simulink model "Feeder_IREQ_2012"  (Simulink 8.3)
settings: Solver=FixedStepDiscrete  StartTime=0.0  StopTime=100  FixedStep=50e-6  RelTol=1e-3
InitFcn:
  | Ts= 50e-6;
undefined symbols (not defined in the file): D11, Delta, DiscIntNeverNeededParam, Ion, kaimal_num, Lithium, u0
libraries: powerlib x62, powerlib_extras x49, simulink x14, simulink_extras x12, sps_avr x2, electricdrivelib x1
(part 3 of 5)

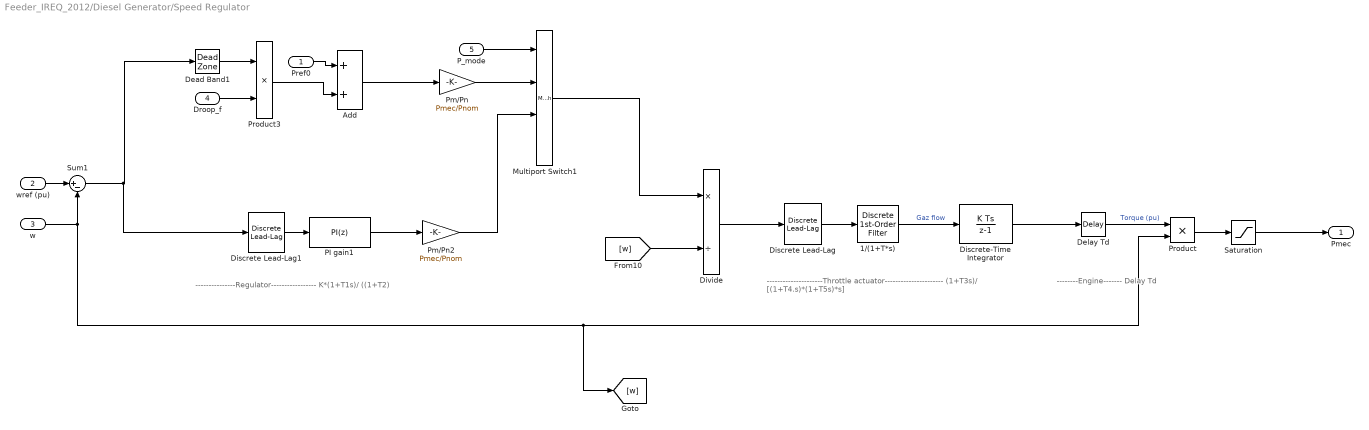
== system Feeder_IREQ_2012/Diesel Generator/Speed Regulator ==
  note: ---------------------Throttle actuator----------------------
      | (1+T3s)/ [(1+T4.s)*(1+T5s)*s]
  note: ---------------Regulator-----------------
      | K*(1+T1s)/ ((1+T2)
  note: --------Engine-------
      | Delay Td
  Pref0 : Inport
  wref (pu) : Inport  Port=2
  w : Inport  Port=3
  Droop_f : Inport  Port=4
  P_mode : Inport  Port=5
  1/(1+T*s) : powerlib_extras/Discrete  Control Blocks/Discrete 1st-Order Filter  FilterType=Lowpass  Tc=Ta(3)  Ts=Ts  Initialize=off  Vac_Init=[0.8 -25 60]  Vdc_Init=-0.4  PlotResponse=off  param1=[1 500 0.1]
  Add : Sum
  Dead Band1 : DeadZone  LowerValue=-0.001  UpperValue=0.001  SaturateOnIntegerOverflow=on
  Delay Td : TransportDelay  DelayTime=Td  InitialOutput=Pm0
  Discrete Lead-Lag : powerlib_extras/Discrete  Control Blocks/Discrete Lead-Lag  T1=Ta(1)  T2=Ta(2)  V_Init=0  Ts=Ts
  Discrete Lead-Lag1 : powerlib_extras/Discrete  Control Blocks/Discrete Lead-Lag  T1=Tr(1)  T2=Tr(2)  V_Init=0  Ts=Ts
  Discrete-Time Integrator : DiscreteIntegrator  InitialCondition=Pm0  SampleTime=Ts  LimitOutput=on  UpperSaturationLimit=Tlim(2)  LowerSaturationLimit=Tlim(1)  ICPrevOutput=DiscIntNeverNeededParam  ICPrevScaledInput=DiscIntNeverNeededParam
  Divide : Product  Inputs=*/
  Multiport Switch1 : MultiPortSwitch  SaturateOnIntegerOverflow=on  InputSameDT=on
  PI gain1 : simulink/Continuous/PID Controller  Controller=PI  TimeDomain=Discrete-time  SampleTime=-1  IntegratorMethod=Forward Euler  FilterMethod=Forward Euler  Form=Parallel  P=100  I=100  D=-14.7932376623781  N=587.187356380874  InitialConditionSource=internal  InitialConditionForIntegrator=0  InitialConditionForFilter=0  ExternalReset=none  LimitOutput=off  UpperSaturationLimit=1.05  LowerSaturationLimit=.95  LinearizeAsGain=off  AntiWindupMode=back-calculation  Kb=1  TrackingMode=off  Kt=1  PParamMin=[]  PParamMax=[]  IParamMin=[]  IParamMax=[]  DParamMin=[]  DParamMax=[]  NParamMin=[]  NParamMax=[]  KbParamMin=[]  KbParamMax=[]  KtParamMin=[]  KtParamMax=[]  POutMin=[]  POutMax=[]  IOutMin=[]  IOutMax=[]  DOutMin=[]  DOutMax=[]  NOutMin=[]  NOutMax=[]  KbOutMin=[]  KbOutMax=[]  KtOutMin=[]  KtOutMax=[]  IntegratorOutMin=[]  IntegratorOutMax=[]  FilterOutMin=[]  FilterOutMax=[]  SumOutMin=[]  SumOutMax=[]  SumI1OutMin=[]  SumI1OutMax=[]  SumI2OutMin=[]  SumI2OutMax=[]  SumI3OutMin=[]  SumI3OutMax=[]  SumDOutMin=[]  SumDOutMax=[]  SaturationOutMin=[]  SaturationOutMax=[]  IntegratorContinuousStateAttributes=''  IntegratorStateMustResolveToSignalObject=off  IntegratorRTWStateStorageClass=Auto  FilterContinuousStateAttributes=''  FilterStateMustResolveToSignalObject=off  FilterRTWStateStorageClass=Auto
  Pm/Pn : Gain  Gain=Pmec/Pnom
  Pm/Pn2 : Gain  Gain=Pmec/Pnom
  Product : Product  SaturateOnIntegerOverflow=on  InputSameDT=on  OutDataTypeStr=Inherit: Same as first input
  Product3 : Product  RndMeth=Zero
  Saturation : Saturate  UpperLimit=Pmec/Pnom  LowerLimit=0
  Sum1 : Sum  Inputs=|+-  SaturateOnIntegerOverflow=on
  Pmec : Outport  InitialOutput=0
  wires:
  wref (pu)/1 -> Sum1/1
  Dead Band1/1 -> Product3/1
  Droop_f/1 -> Product3/2
  Pref0/1 -> Add/1
  Product3/1 -> Add/2
  P_mode/1 -> Multiport Switch1/1
  Add/1 -> Pm/Pn/1
  Pm/Pn/1 -> Multiport Switch1/2
  w/1 -> [w], Product/2, Sum1/2
  Sum1/1 -> Discrete Lead-Lag1/1, Dead Band1/1
  Delay Td/1 -> Product/1  "Torque (pu)"
  Discrete Lead-Lag/1 -> 1/(1+T*s)/1
  1/(1+T*s)/1 -> Discrete-Time Integrator/1  "Gaz flow"
  Discrete Lead-Lag1/1 -> PI gain1/1
  Discrete-Time Integrator/1 -> Delay Td/1
  PI gain1/1 -> Pm/Pn2/1
  [w] -> Divide/2
  Divide/1 -> Discrete Lead-Lag/1
  Saturation/1 -> Pmec/1
  Product/1 -> Saturation/1
  Multiport Switch1/1 -> Divide/1
  Pm/Pn2/1 -> Multiport Switch1/3

== system Feeder_IREQ_2012/Diesel Generator/Voltage Droop with Q ==
  Vref : Inport
  Droop_v : Inport  Port=2
  fixed_Q : Inport  Port=3
  Qpcc : Inport  Port=4
  VPCC : Inport  Port=5
  Dead Band1 : DeadZone  LowerValue=-0.01  UpperValue=0.01  SaturateOnIntegerOverflow=on
  PI1 : simulink/Continuous/PID Controller  Controller=PI  TimeDomain=Discrete-time  SampleTime=-1  IntegratorMethod=Forward Euler  FilterMethod=Forward Euler  Form=Parallel  P=.5  I=5  D=-14.7932376623781  N=587.187356380874  InitialConditionSource=internal  InitialConditionForIntegrator=0  InitialConditionForFilter=0  ExternalReset=none  LimitOutput=on  UpperSaturationLimit=1.05  LowerSaturationLimit=.94  LinearizeAsGain=off  AntiWindupMode=none  Kb=1  TrackingMode=off  Kt=1  PParamMin=[]  PParamMax=[]  IParamMin=[]  IParamMax=[]  DParamMin=[]  DParamMax=[]  NParamMin=[]  NParamMax=[]  KbParamMin=[]  KbParamMax=[]  KtParamMin=[]  KtParamMax=[]  POutMin=[]  POutMax=[]  IOutMin=[]  IOutMax=[]  DOutMin=[]  DOutMax=[]  NOutMin=[]  NOutMax=[]  KbOutMin=[]  KbOutMax=[]  KtOutMin=[]  KtOutMax=[]  IntegratorOutMin=[]  IntegratorOutMax=[]  FilterOutMin=[]  FilterOutMax=[]  SumOutMin=[]  SumOutMax=[]  SumI1OutMin=[]  SumI1OutMax=[]  SumI2OutMin=[]  SumI2OutMax=[]  SumI3OutMin=[]  SumI3OutMax=[]  SumDOutMin=[]  SumDOutMax=[]  SaturationOutMin=[]  SaturationOutMax=[]  IntegratorContinuousStateAttributes=''  IntegratorStateMustResolveToSignalObject=off  IntegratorRTWStateStorageClass=Auto  FilterContinuousStateAttributes=''  FilterStateMustResolveToSignalObject=off  FilterRTWStateStorageClass=Auto
  Product3 : Product  RndMeth=Zero
  Sum1 : Sum  Inputs=+-  SaturateOnIntegerOverflow=on  InputSameDT=on  OutDataTypeStr=Inherit: Same as first input
  Sum2 : Sum  Inputs=+-  SaturateOnIntegerOverflow=on  InputSameDT=on  OutDataTypeStr=Inherit: Same as first input
  Sum4 : Sum  SaturateOnIntegerOverflow=on  InputSameDT=on  OutDataTypeStr=Inherit: Same as first input
  Vf : Outport
  wires:
  Sum2/1 -> Dead Band1/1
  Dead Band1/1 -> Product3/1
  Droop_v/1 -> Product3/2
  Product3/1 -> Sum4/1
  Vref/1 -> Sum2/1
  Qpcc/1 -> Sum1/2
  Sum1/1 -> PI1/1
  PI1/1 -> Vf/1
  fixed_Q/1 -> Sum4/2
  Sum4/1 -> Sum1/1
  VPCC/1 -> Sum2/2

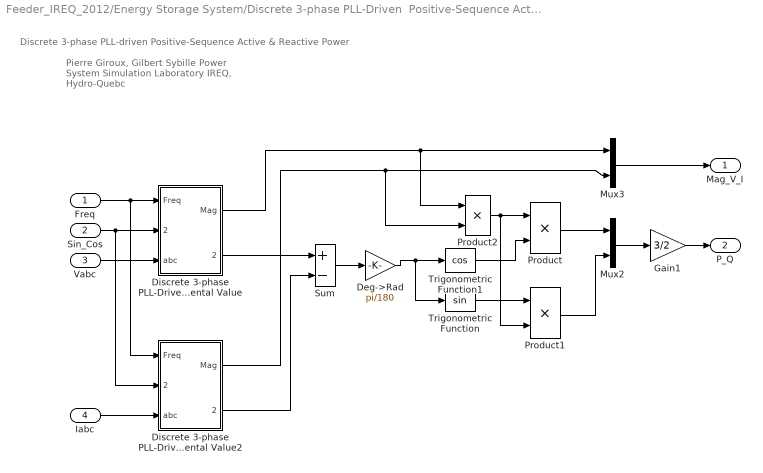
== system Feeder_IREQ_2012/Energy Storage System/Discrete 3-phase PLL-Driven  Positive-Sequence Active & Reactive Power ==
  note: Pierre Giroux, Gilbert Sybille
      | Power System Simulation Laboratory
      | IREQ, Hydro-Quebc
  note: Discrete 3-phase PLL-driven Positive-Sequence Active & Reactive Power
  Freq : Inport  PortDimensions=1
  Sin_Cos : Inport  Port=2  PortDimensions=2
  Vabc : Inport  Port=3  PortDimensions=3
  Iabc : Inport  Port=4  PortDimensions=3
  Deg->Rad : Gain  Gain=pi/180  SaturateOnIntegerOverflow=on  OutDataTypeStr=Inherit: Same as input  ParamDataTypeStr=Inherit: Same as input
  Discrete 3-phase PLL-Driven Positive-Sequence Fundamental Value : Subsystem  mask(Discrete 3-phase PLL-Driven Positive-Sequence Fundamental Value){Finit=Finit, Fmin=Fmin, Par_Init=Par_Vinit, Ts=Ts}
      mask prompts: Finit "Initial frequency (Hz):"; Fmin "Minimum frequency (Hz):"; Par_Init "Initial input (positive component): [ Mag  Phase-relative-to-PLL(degrees) ]"; Ts "Sample time:"
      mask help:
      | For a supplied fundamental frequency (port Freq), this discrete block computes  the positive-sequence component (Magnitude and Phase)  of a set of three balanced or unbalanced signals (port abc) which may contain harmonics.
      |  Input port "Sin_Cos" (a two-dimension signal) provides the reference frame required for the computation..
      |  First and second outputs return respectively the magnitude and phase (in degrees relative to the PLL phase)) of the fundamental.
      | For the first cycle of simulation, the outputs are held constant to the values specified by the parameter "Initial input".
      | constant to the values specified by the parameter "Initial input". The value of the parameter "Minimum frequency" is used to determine the buffer size of the "Variable Transport Delay" block found inside this subsystem.
      mask init:
      | Real_Init=Par_Init(1)*cos(pi/180*Par_Init(2));
      | Imag_Init=Par_Init(1)*sin(pi/180*Par_Init(2));
      | power_initmask();
      settings: OpenFcn=power_openblockproxy();
  Discrete 3-phase PLL-Driven Positive-Sequence Fundamental Value2 : Subsystem  mask(Discrete 3-phase PLL-Driven Positive-Sequence Fundamental Value){Finit=Finit, Fmin=Fmin, Par_Init=Par_Iinit, Ts=Ts}
      mask prompts: Finit "Initial frequency (Hz):"; Fmin "Minimum frequency (Hz):"; Par_Init "Initial input (positive component): [ Mag  Phase-relative-to-PLL(degrees) ]"; Ts "Sample time:"
      mask help:
      | For a supplied fundamental frequency (port Freq), this discrete block computes  the positive-sequence component (Magnitude and Phase)  of a set of three balanced or unbalanced signals (port abc) which may contain harmonics.
      |  Input port "Sin_Cos" (a two-dimension signal) provides the reference frame required for the computation..
      |  First and second outputs return respectively the magnitude and phase (in degrees relative to the PLL phase)) of the fundamental.
      | For the first cycle of simulation, the outputs are held constant to the values specified by the parameter "Initial input".
      | constant to the values specified by the parameter "Initial input". The value of the parameter "Minimum frequency" is used to determine the buffer size of the "Variable Transport Delay" block found inside this subsystem.
      mask init:
      | Real_Init=Par_Init(1)*cos(pi/180*Par_Init(2));
      | Imag_Init=Par_Init(1)*sin(pi/180*Par_Init(2));
      | power_initmask();
      settings: OpenFcn=power_openblockproxy();
  Gain1 : Gain  Gain=3/2  SaturateOnIntegerOverflow=on  OutDataTypeStr=Inherit: Same as input  ParamDataTypeStr=Inherit: Same as input
  Mux2 : Mux  Inputs=2
  Mux3 : Mux  Inputs=2
  Product : Product  SaturateOnIntegerOverflow=on  InputSameDT=on  OutDataTypeStr=Inherit: Same as first input
  Product1 : Product  SaturateOnIntegerOverflow=on  InputSameDT=on  OutDataTypeStr=Inherit: Same as first input
  Product2 : Product  SaturateOnIntegerOverflow=on  InputSameDT=on  OutDataTypeStr=Inherit: Same as first input
  Sum : Sum  Inputs=+-  SaturateOnIntegerOverflow=on  InputSameDT=on  OutDataTypeStr=Inherit: Same as first input
  Trigonometric Function : Trigonometry
  Trigonometric Function1 : Trigonometry  Operator=cos
  Mag_V_I : Outport
  P_Q : Outport  Port=2
  wires:
  Iabc/1 -> Discrete 3-phase PLL-Driven Positive-Sequence Fundamental Value2/3(abc)
  Discrete 3-phase PLL-Driven Positive-Sequence Fundamental Value2/1(Mag) -> Product2/2, Mux3/2
  Product2/1 -> Product1/2, Product/1
  Gain1/1 -> P_Q/1
  Mux3/1 -> Mag_V_I/1
  Product1/1 -> Mux2/2
  Product/1 -> Mux2/1
  Mux2/1 -> Gain1/1
  Trigonometric Function/1 -> Product1/1
  Trigonometric Function1/1 -> Product/2
  Deg->Rad/1 -> Trigonometric Function/1, Trigonometric Function1/1
  Sum/1 -> Deg->Rad/1
  Discrete 3-phase PLL-Driven Positive-Sequence Fundamental Value2/2(Phase) -> Sum/2
  Discrete 3-phase PLL-Driven Positive-Sequence Fundamental Value/1(Mag) -> Product2/1, Mux3/1
  Discrete 3-phase PLL-Driven Positive-Sequence Fundamental Value/2(Phase) -> Sum/1
  Sin_Cos/1 -> Discrete 3-phase PLL-Driven Positive-Sequence Fundamental Value2/2(Sin_Cos), Discrete 3-phase PLL-Driven Positive-Sequence Fundamental Value/2(Sin_Cos)
  Freq/1 -> Discrete 3-phase PLL-Driven Positive-Sequence Fundamental Value2/1(Freq), Discrete 3-phase PLL-Driven Positive-Sequence Fundamental Value/1(Freq)
  Vabc/1 -> Discrete 3-phase PLL-Driven Positive-Sequence Fundamental Value/3(abc)

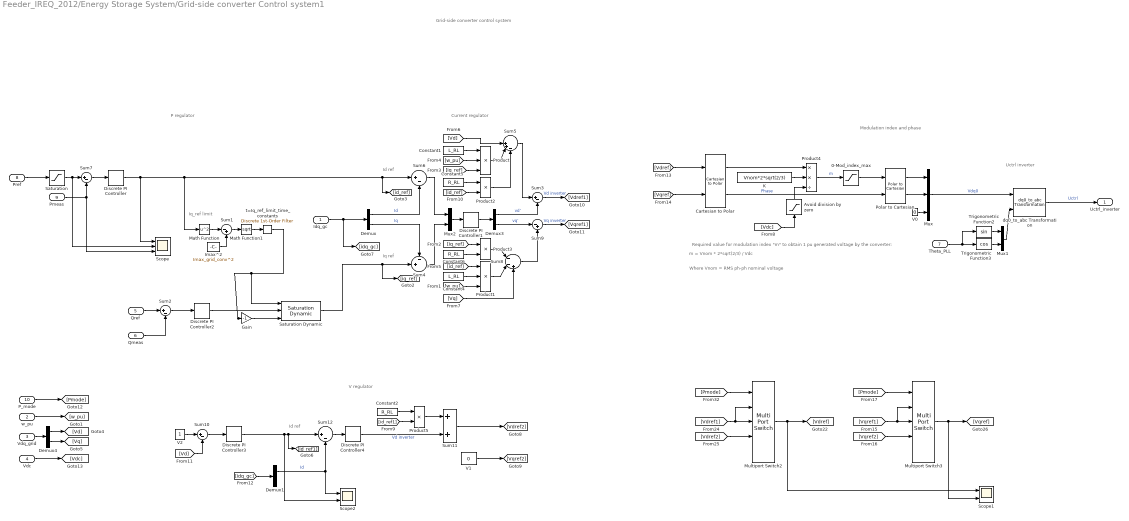
== system Feeder_IREQ_2012/Energy Storage System/Grid-side converter Control system1 ==
  note: Grid-side converter control system
  note: P regulator
  note: Iq_ref limit
  note: Current regulator
  note: Id ref
  note: Iq ref
  note: Required value for modulation index "m" to obtain 1 pu generated voltage by the converter:
  note: m = Vnom * 2*sqrt(2/3) / Vdc
  note: Where Vnom = RMS ph-ph nominal voltage
  note: Modulation index and phase
  note: Uctrl inverter
  note: V regulator
  note: Id ref
  Idq_gc : Inport
  w_pu : Inport  Port=2
  Vdq_grid : Inport  Port=3
  Vdc : Inport  Port=4
  Qref : Inport  Port=5
  Qmeas : Inport  Port=6
  Theta_PLL : Inport  Port=7
  Pref : Inport  Port=8
  Pmeas : Inport  Port=9
  P_mode : Inport  Port=10
  0-Mod_index_max : Saturate  UpperLimit=Mod_index_max  LowerLimit=0
  Avoid division by zero : Saturate  UpperLimit=1e6  LowerLimit=1e-6
  Cartesian to Polar : simulink_extras/Transformations/Cartesian to Polar
  Constant1 : Constant  Value=L_RL
  Constant2 : Constant  Value=R_RL
  Constant4 : Constant  Value=L_RL
  Constant5 : Constant  Value=R_RL
  Constant6 : Constant  Value=R_RL
  Demux{,1,3..4} (4 alike) : Demux  Outputs=2
  Discrete PI Controller : powerlib_extras/Discrete  Control Blocks/Discrete PI Controller  Kp=1  Ki=50  Par_Limits=[1 -1]*Imax_grid_conv  Init=0  Ts=Ts
  Discrete PI Controller1 : powerlib_extras/Discrete  Control Blocks/Discrete PI Controller  Kp=1  Ki=50  Par_Limits=[1 -1]*Current_reg_output_limit  Init=0  Ts=Ts
  Discrete PI Controller2 : powerlib_extras/Discrete  Control Blocks/Discrete PI Controller  Kp=1  Ki=50  Par_Limits=[1 -1]*Imax_grid_conv  Init=0  Ts=Ts
  Discrete PI Controller3 : powerlib_extras/Discrete  Control Blocks/Discrete PI Controller  Kp=1  Ki=10  Par_Limits=[1 -1]*Imax_grid_conv  Init=0  Ts=Ts
  Discrete PI Controller4 : powerlib_extras/Discrete  Control Blocks/Discrete PI Controller  Kp=1  Ki=50  Par_Limits=[1 -1]*Current_reg_output_limit  Init=0  Ts=Ts
  Gain : Gain  Gain=-1  SaturateOnIntegerOverflow=on  OutDataTypeStr=Inherit: Same as input  ParamDataTypeStr=Inherit: Same as input
  Imax^2 : Constant  Value=Imax_grid_conv^2
  K : Constant  Value=Vnom*2*sqrt(2/3)
  Math Function : Math  Operator=square  SaturateOnIntegerOverflow=on
  Math Function1 : Math  Operator=sqrt  SaturateOnIntegerOverflow=on
  Multiport Switch2 : MultiPortSwitch  Inputs=4  SaturateOnIntegerOverflow=on  InputSameDT=on
  Multiport Switch3 : MultiPortSwitch  Inputs=4  SaturateOnIntegerOverflow=on  InputSameDT=on
  Mux : Mux  Inputs=3
  Mux1 : Mux  Inputs=2
  Mux2 : Mux  Inputs=2
  Polar to Cartesian : simulink_extras/Transformations/Polar to Cartesian
  Product : Product  Inputs=3  SaturateOnIntegerOverflow=on  InputSameDT=on  OutDataTypeStr=Inherit: Same as first input
  Product1 : Product  Inputs=3  SaturateOnIntegerOverflow=on  InputSameDT=on  OutDataTypeStr=Inherit: Same as first input
  Product2 : Product  SaturateOnIntegerOverflow=on  InputSameDT=on  OutDataTypeStr=Inherit: Same as first input
  Product3 : Product  SaturateOnIntegerOverflow=on  InputSameDT=on  OutDataTypeStr=Inherit: Same as first input
  Product4 : Product  Inputs=**/  SaturateOnIntegerOverflow=on  InputSameDT=on  OutDataTypeStr=Inherit: Same as first input
  Product5 : Product  SaturateOnIntegerOverflow=on  InputSameDT=on  OutDataTypeStr=Inherit: Same as first input
  Saturation : Saturate  UpperLimit=Pbat/Pnom  LowerLimit=-Pbat/Pnom
  Saturation Dynamic : simulink/Discontinuities/Saturation Dynamic  OutMin=[]  OutMax=[]  OutDataTypeStr=Inherit: Same as second input  OutDataType=fixdt(1, 16)  OutScaling=2^-10  DoSatur=off
  Scope : Scope  NumInputPorts=3
  Scope1 : Scope  NumInputPorts=2
  Scope2 : Scope  NumInputPorts=2
  Sum1 : Sum  Inputs=|-+  SaturateOnIntegerOverflow=on  InputSameDT=on  OutDataTypeStr=Inherit: Same as first input
  Sum{2..3,6..7,10,12} (6 alike) : Sum  Inputs=|+-  SaturateOnIntegerOverflow=on  InputSameDT=on  OutDataTypeStr=Inherit: Same as first input
  Sum11 : Sum  SaturateOnIntegerOverflow=on  InputSameDT=on  OutDataTypeStr=Inherit: Same as first input
  Sum4 : Sum  Inputs=-+|  SaturateOnIntegerOverflow=on  InputSameDT=on  OutDataTypeStr=Inherit: Same as first input
  Sum5 : Sum  Inputs=||++-  SaturateOnIntegerOverflow=on  InputSameDT=on  OutDataTypeStr=Inherit: Same as first input
  Sum8 : Sum  Inputs=|--+  SaturateOnIntegerOverflow=on  InputSameDT=on  OutDataTypeStr=Inherit: Same as first input
  Sum9 : Sum  Inputs=|-+  SaturateOnIntegerOverflow=on  InputSameDT=on  OutDataTypeStr=Inherit: Same as first input
  Trigonometric Function2 : Trigonometry
  Trigonometric Function3 : Trigonometry  Operator=cos
  V0 : Constant  Value=0
  V1 : Constant  Value=0
  V2 : Constant
  dq0_to_abc Transformation : powerlib_extras/Measurements/dq0_to_abc Transformation
  t=Iq_ref_limit_time_constants : powerlib_extras/Discrete  Control Blocks/Discrete 1st-Order Filter  FilterType=Lowpass  Tc=Iq_ref_limit_time_constant  Ts=Ts  Initialize=on  Vac_Init=[0 0 0]  Vdc_Init=Imax_grid_conv  PlotResponse=off  param1=[1 500 0.1]
  Uctrl_inverter : Outport
  wires:
  Vdc/1 -> [Vdc]
  Vdq_grid/1 -> Demux4/1
  Discrete PI Controller/1 -> Math Function/1, Sum6/1, [id_ref], Scope/1
  Qmeas/1 -> Sum2/2
  Sum2/1 -> Discrete PI Controller2/1
  Math Function1/1 -> t=Iq_ref_limit_time_constants/1
  Sum1/1 -> Math Function1/1
  Imax^2/1 -> Sum1/2
  Math Function/1 -> Sum1/1
  t=Iq_ref_limit_time_constants/1 -> Gain/1, Saturation Dynamic/1
  Constant4/1 -> Product1/2
  Discrete PI Controller1/1 -> Demux3/1
  Mux2/1 -> Discrete PI Controller1/1
  Constant1/1 -> Product/1
  Demux/2 -> Sum4/1  "Iq"
  Demux/1 -> Sum6/2  "Id"
  Product/1 -> Sum5/2
  Constant5/1 -> Product2/1
  Constant6/1 -> Product3/2
  Product1/1 -> Sum8/2
  Product2/1 -> Sum5/3
  Product3/1 -> Sum8/1
  Sum6/1 -> Mux2/1
  Sum4/1 -> Mux2/2
  [w_pu] -> Product1/3
  [w_pu] -> Product/2
  [iq_ref] -> Product/3
  [id_ref] -> Product2/2
  [iq_ref] -> Product3/1
  [id_ref] -> Product1/1
  Demux3/1 -> Sum3/2  "vd'"
  Demux3/2 -> Sum9/1  "vq'"
  w_pu/1 -> [w_pu]
  Demux4/1 -> [Vd]
  Demux4/2 -> [Vq]
  [Vq] -> Sum8/3
  [Vd] -> Sum5/1
  Product4/1 -> 0-Mod_index_max/1  "m"
  K/1 -> Product4/2
  Avoid division by zero/1 -> Product4/3
  Cartesian to Polar/1 -> Product4/1
  [Vdc] -> Avoid division by zero/1
  Polar to Cartesian/2 -> Mux/2
  Polar to Cartesian/1 -> Mux/1
  V0/1 -> Mux/3
  Trigonometric Function3/1 -> Mux1/2
  Trigonometric Function2/1 -> Mux1/1
  Mux1/1 -> dq0_to_abc Transformation/2
  Cartesian to Polar/2 -> Polar to Cartesian/2  "Phase"
  Mux/1 -> dq0_to_abc Transformation/1  "Vdq0"
  dq0_to_abc Transformation/1 -> Uctrl_inverter/1  "Uctrl"
  Idq_gc/1 -> [idq_gc], Demux/1
  0-Mod_index_max/1 -> Polar to Cartesian/1
  Sum5/1 -> Sum3/1
  Sum8/1 -> Sum9/2
  Pref/1 -> Saturation/1
  Qref/1 -> Sum2/1
  Gain/1 -> Saturation Dynamic/3
  Discrete PI Controller2/1 -> Saturation Dynamic/2
  Pmeas/1 -> Scope/3, Sum7/2
  Saturation Dynamic/1 -> Sum4/2, [iq_ref]
  Saturation/1 -> Scope/2, Sum7/1
  Sum7/1 -> Discrete PI Controller/1
  Theta_PLL/1 -> Trigonometric Function2/1, Trigonometric Function3/1
  Discrete PI Controller3/1 -> Scope2/2, Sum12/1, [id_ref1]
  Demux1/1 -> Scope2/1, Sum12/2  "Id"
  Constant2/1 -> Product5/1
  Sum12/1 -> Discrete PI Controller4/1
  [id_ref1] -> Product5/2
  Discrete PI Controller4/1 -> Sum11/2  "Vd inverter"
  V2/1 -> Sum10/1
  Sum10/1 -> Discrete PI Controller3/1
  [Vd] -> Sum10/2
  Sum11/1 -> [Vdref2]
  Product5/1 -> Sum11/1
  [idq_gc] -> Demux1/1
  [Pmode] -> Multiport Switch2/1
  [Pmode] -> Multiport Switch3/1
  Multiport Switch2/1 -> Scope1/1, [Vdref]
  Multiport Switch3/1 -> Scope1/2, [Vqref]
  V1/1 -> [Vqref2]
  Sum3/1 -> [Vdref1]  "Vd inverter"
  Sum9/1 -> [Vqref1]  "Vq inverter"
  P_mode/1 -> [Pmode]
  [Vqref2] -> Multiport Switch3/4
  [Vdref1] -> Multiport Switch2/2, Multiport Switch2/3
  [Vdref2] -> Multiport Switch2/4
  [Vqref1] -> Multiport Switch3/2, Multiport Switch3/3
  [Vdref] -> Cartesian to Polar/1
  [Vqref] -> Cartesian to Polar/2

== system Feeder_IREQ_2012/Energy Storage System/Reactive power gain1 ==
  In1 : Inport
  Product : Product  RndMeth=Zero
  Product1 : Product  RndMeth=Zero
  Sign : Signum
  Trigonometric Function1 : Trigonometry  Operator=acos
  Trigonometric Function2 : Trigonometry  Operator=tan
  Out1 : Outport
  wires:
  In1/1 -> Sign/1, Product/2
  Sign/1 -> Product/1, Product1/1
  Product/1 -> Trigonometric Function1/1
  Trigonometric Function1/1 -> Product1/2
  Product1/1 -> Trigonometric Function2/1
  Trigonometric Function2/1 -> Out1/1

== system Feeder_IREQ_2012/Energy Storage System/Speed Regulator ==
  Pref0 : Inport
  wref (pu) : Inport  Port=2
  w : Inport  Port=3
  Droop_f : Inport  Port=4
  P_mode : Inport  Port=5
  Add : Sum
  Dead Band1 : DeadZone  LowerValue=-0.001  UpperValue=0.001  SaturateOnIntegerOverflow=on
  Multiport Switch1 : MultiPortSwitch  Inputs=4  SaturateOnIntegerOverflow=on  InputSameDT=on
  PI gain : simulink/Continuous/PID Controller  Controller=PI  TimeDomain=Discrete-time  SampleTime=-1  IntegratorMethod=Trapezoidal  FilterMethod=Forward Euler  Form=Parallel  P=30  I=30  D=-14.7932376623781  N=587.187356380874  InitialConditionSource=internal  InitialConditionForIntegrator=0  InitialConditionForFilter=0  ExternalReset=none  LimitOutput=off  UpperSaturationLimit=Pbat/Pnom  LowerSaturationLimit=-Pbat/Pnom  LinearizeAsGain=off  AntiWindupMode=back-calculation  Kb=1  TrackingMode=off  Kt=1  PParamMin=[]  PParamMax=[]  IParamMin=[]  IParamMax=[]  DParamMin=[]  DParamMax=[]  NParamMin=[]  NParamMax=[]  KbParamMin=[]  KbParamMax=[]  KtParamMin=[]  KtParamMax=[]  POutMin=[]  POutMax=[]  IOutMin=[]  IOutMax=[]  DOutMin=[]  DOutMax=[]  NOutMin=[]  NOutMax=[]  KbOutMin=[]  KbOutMax=[]  KtOutMin=[]  KtOutMax=[]  IntegratorOutMin=[]  IntegratorOutMax=[]  FilterOutMin=[]  FilterOutMax=[]  SumOutMin=[]  SumOutMax=[]  SumI1OutMin=[]  SumI1OutMax=[]  SumI2OutMin=[]  SumI2OutMax=[]  SumI3OutMin=[]  SumI3OutMax=[]  SumDOutMin=[]  SumDOutMax=[]  SaturationOutMin=[]  SaturationOutMax=[]  IntegratorContinuousStateAttributes=''  IntegratorStateMustResolveToSignalObject=off  IntegratorRTWStateStorageClass=Auto  FilterContinuousStateAttributes=''  FilterStateMustResolveToSignalObject=off  FilterRTWStateStorageClass=Auto
  Pbat/Pnom1 : Gain  Gain=Pbat/Pnom
  Product3 : Product  RndMeth=Zero
  Saturation : Saturate  UpperLimit=Pbat/Pnom  LowerLimit=-Pbat/Pnom
  Scope : Scope  NumInputPorts=2
  Sum1 : Sum  Inputs=|+-  SaturateOnIntegerOverflow=on
  Pbat : Outport  InitialOutput=0
  wires:
  w/1 -> Sum1/2
  Multiport Switch1/1 -> Saturation/1
  wref (pu)/1 -> Sum1/1
  Sum1/1 -> Scope/2, Dead Band1/1, PI gain/1
  Dead Band1/1 -> Product3/1
  Droop_f/1 -> Product3/2
  Pref0/1 -> Add/1
  Product3/1 -> Add/2
  P_mode/1 -> Multiport Switch1/1
  Add/1 -> Pbat/Pnom1/1
  Saturation/1 -> Scope/1, Pbat/1
  Pbat/Pnom1/1 -> Multiport Switch1/2
  PI gain/1 -> Multiport Switch1/3

== system Feeder_IREQ_2012/RDER/Discrete 3-phase PLL-Driven  Positive-Sequence Active & Reactive Power ==
  note: Pierre Giroux, Gilbert Sybille
      | Power System Simulation Laboratory
      | IREQ, Hydro-Quebc
  note: Discrete 3-phase PLL-driven Positive-Sequence Active & Reactive Power
  Freq : Inport  PortDimensions=1
  Sin_Cos : Inport  Port=2  PortDimensions=2
  Vabc : Inport  Port=3  PortDimensions=3
  Iabc : Inport  Port=4  PortDimensions=3
  Deg->Rad : Gain  Gain=pi/180  SaturateOnIntegerOverflow=on  OutDataTypeStr=Inherit: Same as input  ParamDataTypeStr=Inherit: Same as input
  Discrete 3-phase PLL-Driven Positive-Sequence Fundamental Value : Subsystem  mask(Discrete 3-phase PLL-Driven Positive-Sequence Fundamental Value){Finit=Finit, Fmin=Fmin, Par_Init=Par_Vinit, Ts=Ts}
      mask prompts: Finit "Initial frequency (Hz):"; Fmin "Minimum frequency (Hz):"; Par_Init "Initial input (positive component): [ Mag  Phase-relative-to-PLL(degrees) ]"; Ts "Sample time:"
      mask help:
      | For a supplied fundamental frequency (port Freq), this discrete block computes  the positive-sequence component (Magnitude and Phase)  of a set of three balanced or unbalanced signals (port abc) which may contain harmonics.
      |  Input port "Sin_Cos" (a two-dimension signal) provides the reference frame required for the computation..
      |  First and second outputs return respectively the magnitude and phase (in degrees relative to the PLL phase)) of the fundamental.
      | For the first cycle of simulation, the outputs are held constant to the values specified by the parameter "Initial input".
      | constant to the values specified by the parameter "Initial input". The value of the parameter "Minimum frequency" is used to determine the buffer size of the "Variable Transport Delay" block found inside this subsystem.
      mask init:
      | Real_Init=Par_Init(1)*cos(pi/180*Par_Init(2));
      | Imag_Init=Par_Init(1)*sin(pi/180*Par_Init(2));
      | power_initmask();
      settings: OpenFcn=power_openblockproxy();
  Discrete 3-phase PLL-Driven Positive-Sequence Fundamental Value2 : Subsystem  mask(Discrete 3-phase PLL-Driven Positive-Sequence Fundamental Value){Finit=Finit, Fmin=Fmin, Par_Init=Par_Iinit, Ts=Ts}
      mask prompts: Finit "Initial frequency (Hz):"; Fmin "Minimum frequency (Hz):"; Par_Init "Initial input (positive component): [ Mag  Phase-relative-to-PLL(degrees) ]"; Ts "Sample time:"
      mask help:
      | For a supplied fundamental frequency (port Freq), this discrete block computes  the positive-sequence component (Magnitude and Phase)  of a set of three balanced or unbalanced signals (port abc) which may contain harmonics.
      |  Input port "Sin_Cos" (a two-dimension signal) provides the reference frame required for the computation..
      |  First and second outputs return respectively the magnitude and phase (in degrees relative to the PLL phase)) of the fundamental.
      | For the first cycle of simulation, the outputs are held constant to the values specified by the parameter "Initial input".
      | constant to the values specified by the parameter "Initial input". The value of the parameter "Minimum frequency" is used to determine the buffer size of the "Variable Transport Delay" block found inside this subsystem.
      mask init:
      | Real_Init=Par_Init(1)*cos(pi/180*Par_Init(2));
      | Imag_Init=Par_Init(1)*sin(pi/180*Par_Init(2));
      | power_initmask();
      settings: OpenFcn=power_openblockproxy();
  Gain1 : Gain  Gain=3/2  SaturateOnIntegerOverflow=on  OutDataTypeStr=Inherit: Same as input  ParamDataTypeStr=Inherit: Same as input
  Mux2 : Mux  Inputs=2
  Mux3 : Mux  Inputs=2
  Product : Product  SaturateOnIntegerOverflow=on  InputSameDT=on  OutDataTypeStr=Inherit: Same as first input
  Product1 : Product  SaturateOnIntegerOverflow=on  InputSameDT=on  OutDataTypeStr=Inherit: Same as first input
  Product2 : Product  SaturateOnIntegerOverflow=on  InputSameDT=on  OutDataTypeStr=Inherit: Same as first input
  Sum : Sum  Inputs=+-  SaturateOnIntegerOverflow=on  InputSameDT=on  OutDataTypeStr=Inherit: Same as first input
  Trigonometric Function : Trigonometry
  Trigonometric Function1 : Trigonometry  Operator=cos
  Mag_V_I : Outport
  P_Q : Outport  Port=2
  wires:
  Iabc/1 -> Discrete 3-phase PLL-Driven Positive-Sequence Fundamental Value2/3(abc)
  Discrete 3-phase PLL-Driven Positive-Sequence Fundamental Value2/1(Mag) -> Product2/2, Mux3/2
  Product2/1 -> Product1/2, Product/1
  Gain1/1 -> P_Q/1
  Mux3/1 -> Mag_V_I/1
  Product1/1 -> Mux2/2
  Product/1 -> Mux2/1
  Mux2/1 -> Gain1/1
  Trigonometric Function/1 -> Product1/1
  Trigonometric Function1/1 -> Product/2
  Deg->Rad/1 -> Trigonometric Function/1, Trigonometric Function1/1
  Sum/1 -> Deg->Rad/1
  Discrete 3-phase PLL-Driven Positive-Sequence Fundamental Value2/2(Phase) -> Sum/2
  Discrete 3-phase PLL-Driven Positive-Sequence Fundamental Value/1(Mag) -> Product2/1, Mux3/1
  Discrete 3-phase PLL-Driven Positive-Sequence Fundamental Value/2(Phase) -> Sum/1
  Sin_Cos/1 -> Discrete 3-phase PLL-Driven Positive-Sequence Fundamental Value2/2(Sin_Cos), Discrete 3-phase PLL-Driven Positive-Sequence Fundamental Value/2(Sin_Cos)
  Freq/1 -> Discrete 3-phase PLL-Driven Positive-Sequence Fundamental Value2/1(Freq), Discrete 3-phase PLL-Driven Positive-Sequence Fundamental Value/1(Freq)
  Vabc/1 -> Discrete 3-phase PLL-Driven Positive-Sequence Fundamental Value/3(abc)

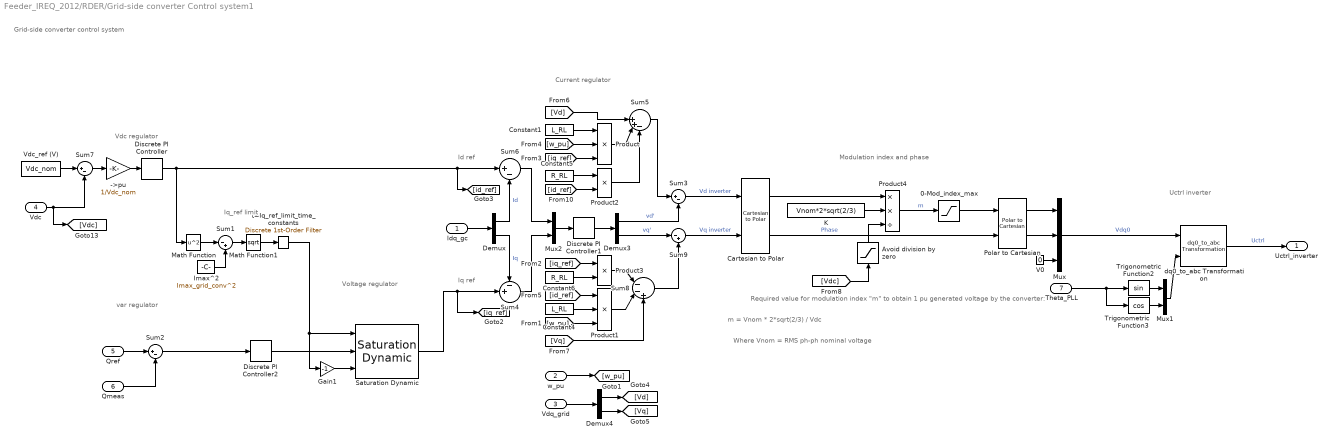
== system Feeder_IREQ_2012/RDER/Grid-side converter Control system1 ==
  note: Grid-side converter control system
  note: var regulator
  note: Voltage regulator
  note: Vdc regulator
  note: Iq_ref limit
  note: Current regulator
  note: Id ref
  note: Iq ref
  note: Required value for modulation index "m" to obtain 1 pu generated voltage by the converter:
  note: m = Vnom * 2*sqrt(2/3) / Vdc
  note: Where Vnom = RMS ph-ph nominal voltage
  note: Modulation index and phase
  note: Uctrl inverter
  Idq_gc : Inport
  w_pu : Inport  Port=2
  Vdq_grid : Inport  Port=3
  Vdc : Inport  Port=4
  Qref : Inport  Port=5
  Qmeas : Inport  Port=6
  Theta_PLL : Inport  Port=7
  ->pu : Gain  Gain=1/Vdc_nom
  0-Mod_index_max : Saturate  UpperLimit=Mod_index_max  LowerLimit=0
  Avoid division by zero : Saturate  UpperLimit=1e6  LowerLimit=1e-6
  Cartesian to Polar : simulink_extras/Transformations/Cartesian to Polar
  Constant1 : Constant  Value=L_RL
  Constant4 : Constant  Value=L_RL
  Constant5 : Constant  Value=R_RL
  Constant6 : Constant  Value=R_RL
  Demux : Demux  Outputs=2
  Demux3 : Demux  Outputs=2
  Demux4 : Demux  Outputs=2
  Discrete PI Controller : powerlib_extras/Discrete  Control Blocks/Discrete PI Controller  Kp=Kp_dc  Ki=Ki_dc  Par_Limits=[1 -1]*Imax_grid_conv  Init=0  Ts=Ts
  Discrete PI Controller1 : powerlib_extras/Discrete  Control Blocks/Discrete PI Controller  Kp=Kp_grid_side_cur_reg  Ki=Ki_grid_side_cur_reg  Par_Limits=[1 -1]*Current_reg_output_limit  Init=0  Ts=Ts
  Discrete PI Controller2 : powerlib_extras/Discrete  Control Blocks/Discrete PI Controller  Kp=1  Ki=10  Par_Limits=[inf -inf]  Init=0  Ts=Ts
  Gain1 : Gain  Gain=-1  SaturateOnIntegerOverflow=on  OutDataTypeStr=Inherit: Same as input  ParamDataTypeStr=Inherit: Same as input
  Imax^2 : Constant  Value=Imax_grid_conv^2
  K : Constant  Value=Vnom*2*sqrt(2/3)
  Math Function : Math  Operator=square  SaturateOnIntegerOverflow=on
  Math Function1 : Math  Operator=sqrt  SaturateOnIntegerOverflow=on
  Mux : Mux  Inputs=3
  Mux1 : Mux  Inputs=2
  Mux2 : Mux  Inputs=2
  Polar to Cartesian : simulink_extras/Transformations/Polar to Cartesian
  Product : Product  Inputs=3  SaturateOnIntegerOverflow=on  InputSameDT=on  OutDataTypeStr=Inherit: Same as first input
  Product1 : Product  Inputs=3  SaturateOnIntegerOverflow=on  InputSameDT=on  OutDataTypeStr=Inherit: Same as first input
  Product2 : Product  SaturateOnIntegerOverflow=on  InputSameDT=on  OutDataTypeStr=Inherit: Same as first input
  Product3 : Product  SaturateOnIntegerOverflow=on  InputSameDT=on  OutDataTypeStr=Inherit: Same as first input
  Product4 : Product  Inputs=**/  SaturateOnIntegerOverflow=on  InputSameDT=on  OutDataTypeStr=Inherit: Same as first input
  Saturation Dynamic : simulink/Discontinuities/Saturation Dynamic  OutMin=[]  OutMax=[]  OutDataTypeStr=Inherit: Same as second input  OutDataType=fixdt(1, 16)  OutScaling=2^-10  DoSatur=off
  Sum1 : Sum  Inputs=|-+  SaturateOnIntegerOverflow=on  InputSameDT=on  OutDataTypeStr=Inherit: Same as first input
  Sum{2..3,6..7} (4 alike) : Sum  Inputs=|+-  SaturateOnIntegerOverflow=on  InputSameDT=on  OutDataTypeStr=Inherit: Same as first input
  Sum4 : Sum  Inputs=-+|  SaturateOnIntegerOverflow=on  InputSameDT=on  OutDataTypeStr=Inherit: Same as first input
  Sum5 : Sum  Inputs=||++-  SaturateOnIntegerOverflow=on  InputSameDT=on  OutDataTypeStr=Inherit: Same as first input
  Sum8 : Sum  Inputs=|--+  SaturateOnIntegerOverflow=on  InputSameDT=on  OutDataTypeStr=Inherit: Same as first input
  Sum9 : Sum  Inputs=|-+  SaturateOnIntegerOverflow=on  InputSameDT=on  OutDataTypeStr=Inherit: Same as first input
  Trigonometric Function2 : Trigonometry
  Trigonometric Function3 : Trigonometry  Operator=cos
  V0 : Constant  Value=0
  Vdc_ref (V) : Constant  Value=Vdc_nom
  dq0_to_abc Transformation : powerlib_extras/Measurements/dq0_to_abc Transformation
  t=Iq_ref_limit_time_constants : powerlib_extras/Discrete  Control Blocks/Discrete 1st-Order Filter  FilterType=Lowpass  Tc=Iq_ref_limit_time_constant  Ts=Ts  Initialize=on  Vac_Init=[0 0 0]  Vdc_Init=Imax_grid_conv  PlotResponse=off  param1=[1 500 0.1]
  Uctrl_inverter : Outport
  wires:
  Vdc/1 -> [Vdc], Sum7/2
  Vdq_grid/1 -> Demux4/1
  Idq_gc/1 -> Demux/1
  Vdc_ref (V)/1 -> Sum7/1
  Sum7/1 -> ->pu/1
  ->pu/1 -> Discrete PI Controller/1
  Discrete PI Controller/1 -> Math Function/1, [id_ref], Sum6/1
  Qmeas/1 -> Sum2/2
  Qref/1 -> Sum2/1
  Math Function1/1 -> t=Iq_ref_limit_time_constants/1
  Sum1/1 -> Math Function1/1
  Imax^2/1 -> Sum1/2
  Math Function/1 -> Sum1/1
  Constant4/1 -> Product1/2
  Discrete PI Controller1/1 -> Demux3/1
  Mux2/1 -> Discrete PI Controller1/1
  Constant1/1 -> Product/1
  Demux/2 -> Sum4/1  "Iq"
  Demux/1 -> Sum6/2  "Id"
  Product/1 -> Sum5/2
  Constant5/1 -> Product2/1
  Constant6/1 -> Product3/2
  Product1/1 -> Sum8/2
  Product2/1 -> Sum5/3
  Product3/1 -> Sum8/1
  Sum6/1 -> Mux2/1
  Sum4/1 -> Mux2/2
  [w_pu] -> Product1/3
  [w_pu] -> Product/2
  [iq_ref] -> Product/3
  [id_ref] -> Product2/2
  [iq_ref] -> Product3/1
  [id_ref] -> Product1/1
  Demux3/1 -> Sum3/2  "vd'"
  Demux3/2 -> Sum9/1  "vq'"
  Sum5/1 -> Sum3/1
  Sum8/1 -> Sum9/2
  w_pu/1 -> [w_pu]
  Demux4/1 -> [Vd]
  Demux4/2 -> [Vq]
  [Vq] -> Sum8/3
  [Vd] -> Sum5/1
  Saturation Dynamic/1 -> Sum4/2, [iq_ref]
  Product4/1 -> 0-Mod_index_max/1  "m"
  K/1 -> Product4/2
  Avoid division by zero/1 -> Product4/3
  Cartesian to Polar/1 -> Product4/1
  [Vdc] -> Avoid division by zero/1
  Sum3/1 -> Cartesian to Polar/1  "Vd inverter"
  Sum9/1 -> Cartesian to Polar/2  "Vq inverter"
  Polar to Cartesian/2 -> Mux/2
  Polar to Cartesian/1 -> Mux/1
  V0/1 -> Mux/3
  Trigonometric Function3/1 -> Mux1/2
  Trigonometric Function2/1 -> Mux1/1
  Mux1/1 -> dq0_to_abc Transformation/2
  0-Mod_index_max/1 -> Polar to Cartesian/1
  Cartesian to Polar/2 -> Polar to Cartesian/2  "Phase"
  Mux/1 -> dq0_to_abc Transformation/1  "Vdq0"
  dq0_to_abc Transformation/1 -> Uctrl_inverter/1  "Uctrl"
  Discrete PI Controller2/1 -> Saturation Dynamic/2
  Gain1/1 -> Saturation Dynamic/3
  t=Iq_ref_limit_time_constants/1 -> Saturation Dynamic/1, Gain1/1
  Sum2/1 -> Discrete PI Controller2/1
  Theta_PLL/1 -> Trigonometric Function3/1, Trigonometric Function2/1

== system Feeder_IREQ_2012/RDER/Reactive power gain1 ==
  In1 : Inport
  Product : Product  RndMeth=Zero
  Product1 : Product  RndMeth=Zero
  Sign : Signum
  Trigonometric Function1 : Trigonometry  Operator=acos
  Trigonometric Function2 : Trigonometry  Operator=tan
  Out1 : Outport
  wires:
  In1/1 -> Sign/1, Product/2
  Sign/1 -> Product/1, Product1/1
  Product/1 -> Trigonometric Function1/1
  Trigonometric Function1/1 -> Product1/2
  Product1/1 -> Trigonometric Function2/1
  Trigonometric Function2/1 -> Out1/1

== system Feeder_IREQ_2012/RDER/Solar Power Emulator ==
  Solar Irrandiance kW/m2 : Inport
  P_avail=f(irr) Canadian Solar CS5P-220M : Lookup  InputValues=irr  Table=P
      mask init:
      | P=[3.78183511444349,12.6357625746008,22.7224915395773,33.3048223622689,44.1901948496012,55.2895875134789,66.5516289225875,77.9428968738727,89.4398972633120,101.025227722755,112.685490819134,124.410048087945,136.190223801743,148.018856018603,159.889894224541,171.798178397444,183.739262423512,195.709242100190,207.704697803349,219.720420522000];
      | irr = [0.05:.05:1];
  Pnom/pu : Gain  Gain=1/219.72
  Saturation : Saturate  UpperLimit=1  LowerLimit=0
  Solar Power : Outport
  wires:
  P_avail=f(irr) Canadian Solar CS5P-220M/1 -> Pnom/pu/1
  Solar Irrandiance kW/m2/1 -> P_avail=f(irr) Canadian Solar CS5P-220M/1
  Pnom/pu/1 -> Saturation/1
  Saturation/1 -> Solar Power/1

== system Feeder_IREQ_2012/RDER/Wind Power Emulator1 ==
  Wind Speed : Inport
  P_avail=f(wind) Enercon E33 : Lookup  InputValues=[1;2;3;4;5;6;7;8;9;10;11;12;13;14;15;16;17;18;19;20;21;22;23;24;25;]  Table=[0;0;5;13.7000000000000;30;55;92;138;196;250;292.800000000000;320;335;335;335;335;335;335;335;335;335;335;335;335;335;]
      mask init:
      | lambda_opt=9.15;        % Optimal lamda in the rotor characteristics
      | Cp_max=0.4788;          % Optimal Cp in the rotor characteristics
      | R_pale=40;              % wind turbine rotor radius [m]
      | S_pale=pi*R_pale^2;     % area swepped by the blades [m^2]
      | ro_air=1.224;           % Air density at 15degC
      | % *****************************************************************
      | % 			 	Wind turbine global characteristics 
      | % *****************************************************************
      | 
      | NumberOfUnits=1;        % Number of units represented by the WT when aggregating
      | Pmec=2e6;               % Nominal mechanical power (W)
      | P_mec = Pmec;
      | 
      | % *****************************************************************
      | % 			 	Generator characteristics 
      | % *****************************************************************
      | 
      | Fnom=60;                %Hz
      | p=3;                    %Number of pairs of poles 
      | w_nom = 2*pi*Fnom/(p);    % Nominal speed for generator [rad/s]
      | % *****************************************************************
      | % 			 	Drive train characteristics 
      | % *****************************************************************
      | 
      | w_nom_wt=188.5/105;         % Nominal rotor speed on low speed side
      | 
      | K_gb =w_nom/w_nom_wt;              % Gearbox Ratio
      | 
      | omega_max = w_nom*1.025;    % maximum rotor speed [rad/s]
      |                             % We allow a 2.5% over synchronous speed before
      |                             % the torque controller reacts.
      | %*****************************************************************
      | %        Power setpoints as a function of rotor speed
      | %        Used for Type "A" control
      | %*****************************************************************
      | 
      | % These points are for Zone_1
      | v_vent_tab_pv =      4 : 0.05 : 7.85;
      | omega_tab_pv =       (v_vent_tab_pv*lambda_opt)/R_pale;
      | P_setpoint_tab_pv =  v_vent_tab_pv.^3*ro_air*pi*R_pale^2*Cp_max*0.5;
      | 
      | % This is the point at the intersection of zone 2 and zone 3
      | v_vent_tab_pv(length(v_vent_tab_pv) +1) = 11.636;
      | omega_tab_pv(length(omega_tab_pv) +1) = omega_max / K_gb;
      | P_setpoint_tab_pv(length(P_setpoint_tab_pv) +1) = P_mec;
      | 
      | % This is the last point for continuity at the end of zone 3
      | v_vent_tab_pv(length(v_vent_tab_pv) +1) = 30;
      | omega_tab_pv(length(omega_tab_pv) +1) = omega_max*2 / K_gb;
      | P_setpoint_tab_pv(length(P_setpoint_tab_pv) +1) = P_mec;
      | 
      | % Added points for stopped operation
      | v_vent_tab_pv2 = [0 3.99 v_vent_tab_pv;];
      | P_setpoint_tab_pv2 = [0 0 P_setpoint_tab_pv;];
  Pnom/pu : Gain  Gain=1/335
  Saturation : Saturate  UpperLimit=1  LowerLimit=0
  Wind Power : Outport
  wires:
  P_avail=f(wind) Enercon E33/1 -> Pnom/pu/1
  Wind Speed/1 -> P_avail=f(wind) Enercon E33/1
  Pnom/pu/1 -> Saturation/1
  Saturation/1 -> Wind Power/1

== system Feeder_IREQ_2012/Rotating Synchronous Machine/Reactive power gain1 ==
  In1 : Inport
  Product : Product  RndMeth=Zero
  Product1 : Product  RndMeth=Zero
  Sign : Signum
  Trigonometric Function1 : Trigonometry  Operator=acos
  Trigonometric Function2 : Trigonometry  Operator=tan
  Out1 : Outport
  wires:
  In1/1 -> Sign/1, Product/2
  Sign/1 -> Product/1, Product1/1
  Product/1 -> Trigonometric Function1/1
  Trigonometric Function1/1 -> Product1/2
  Product1/1 -> Trigonometric Function2/1
  Trigonometric Function2/1 -> Out1/1

== system Feeder_IREQ_2012/Rotating Synchronous Machine/Speed Regulator ==
  Pref0 : Inport
  wref (pu) : Inport  Port=2
  w : Inport  Port=3
  Droop_f : Inport  Port=4
  P_mode : Inport  Port=5
  Add : Sum
  Dead Band1 : DeadZone  LowerValue=-0.001  UpperValue=0.001  SaturateOnIntegerOverflow=on
  Multiport Switch1 : MultiPortSwitch  SaturateOnIntegerOverflow=on  InputSameDT=on
  PI gain : simulink/Continuous/PID Controller  Controller=PI  TimeDomain=Discrete-time  SampleTime=-1  IntegratorMethod=Forward Euler  FilterMethod=Forward Euler  Form=Parallel  P=100  I=100  D=-14.7932376623781  N=587.187356380874  InitialConditionSource=internal  InitialConditionForIntegrator=0  InitialConditionForFilter=0  ExternalReset=none  LimitOutput=off  UpperSaturationLimit=1.05  LowerSaturationLimit=.95  LinearizeAsGain=off  AntiWindupMode=back-calculation  Kb=1  TrackingMode=off  Kt=1  PParamMin=[]  PParamMax=[]  IParamMin=[]  IParamMax=[]  DParamMin=[]  DParamMax=[]  NParamMin=[]  NParamMax=[]  KbParamMin=[]  KbParamMax=[]  KtParamMin=[]  KtParamMax=[]  POutMin=[]  POutMax=[]  IOutMin=[]  IOutMax=[]  DOutMin=[]  DOutMax=[]  NOutMin=[]  NOutMax=[]  KbOutMin=[]  KbOutMax=[]  KtOutMin=[]  KtOutMax=[]  IntegratorOutMin=[]  IntegratorOutMax=[]  FilterOutMin=[]  FilterOutMax=[]  SumOutMin=[]  SumOutMax=[]  SumI1OutMin=[]  SumI1OutMax=[]  SumI2OutMin=[]  SumI2OutMax=[]  SumI3OutMin=[]  SumI3OutMax=[]  SumDOutMin=[]  SumDOutMax=[]  SaturationOutMin=[]  SaturationOutMax=[]  IntegratorContinuousStateAttributes=''  IntegratorStateMustResolveToSignalObject=off  IntegratorRTWStateStorageClass=Auto  FilterContinuousStateAttributes=''  FilterStateMustResolveToSignalObject=off  FilterRTWStateStorageClass=Auto
  Pm/Pn : Gain  Gain=Pmec/Pnom
  Pm/Pn1 : Gain  Gain=Pmec/Pnom
  Product3 : Product  RndMeth=Zero
  Saturation : Saturate  UpperLimit=Pmec/Pnom  LowerLimit=0
  Scope : Scope  NumInputPorts=3
  Sum1 : Sum  Inputs=|+-  SaturateOnIntegerOverflow=on
  Pmec : Outport  InitialOutput=0
  wires:
  w/1 -> Sum1/2
  Multiport Switch1/1 -> Saturation/1
  wref (pu)/1 -> Sum1/1
  Dead Band1/1 -> Product3/1
  Droop_f/1 -> Product3/2
  Pref0/1 -> Add/1
  Product3/1 -> Add/2
  PI gain/1 -> Pm/Pn1/1
  P_mode/1 -> Multiport Switch1/1
  Add/1 -> Pm/Pn/1
  Saturation/1 -> Scope/1, Pmec/1
  Sum1/1 -> Scope/3, PI gain/1, Dead Band1/1
  Pm/Pn/1 -> Multiport Switch1/2
  Pm/Pn1/1 -> Scope/2, Multiport Switch1/3

== system Feeder_IREQ_2012/Rotating Synchronous Machine/Voltage Droop with Q ==
  Vref : Inport
  Droop_v : Inport  Port=2
  fixed_Q : Inport  Port=3
  Qpcc : Inport  Port=4
  VPCC : Inport  Port=5
  Dead Band1 : DeadZone  LowerValue=-0.01  UpperValue=0.01  SaturateOnIntegerOverflow=on
  PI1 : simulink/Continuous/PID Controller  Controller=PI  TimeDomain=Discrete-time  SampleTime=-1  IntegratorMethod=Forward Euler  FilterMethod=Forward Euler  Form=Parallel  P=.5  I=5  D=-14.7932376623781  N=587.187356380874  InitialConditionSource=internal  InitialConditionForIntegrator=0  InitialConditionForFilter=0  ExternalReset=none  LimitOutput=on  UpperSaturationLimit=1.05  LowerSaturationLimit=.94  LinearizeAsGain=off  AntiWindupMode=none  Kb=1  TrackingMode=off  Kt=1  PParamMin=[]  PParamMax=[]  IParamMin=[]  IParamMax=[]  DParamMin=[]  DParamMax=[]  NParamMin=[]  NParamMax=[]  KbParamMin=[]  KbParamMax=[]  KtParamMin=[]  KtParamMax=[]  POutMin=[]  POutMax=[]  IOutMin=[]  IOutMax=[]  DOutMin=[]  DOutMax=[]  NOutMin=[]  NOutMax=[]  KbOutMin=[]  KbOutMax=[]  KtOutMin=[]  KtOutMax=[]  IntegratorOutMin=[]  IntegratorOutMax=[]  FilterOutMin=[]  FilterOutMax=[]  SumOutMin=[]  SumOutMax=[]  SumI1OutMin=[]  SumI1OutMax=[]  SumI2OutMin=[]  SumI2OutMax=[]  SumI3OutMin=[]  SumI3OutMax=[]  SumDOutMin=[]  SumDOutMax=[]  SaturationOutMin=[]  SaturationOutMax=[]  IntegratorContinuousStateAttributes=''  IntegratorStateMustResolveToSignalObject=off  IntegratorRTWStateStorageClass=Auto  FilterContinuousStateAttributes=''  FilterStateMustResolveToSignalObject=off  FilterRTWStateStorageClass=Auto
  Product3 : Product  RndMeth=Zero
  Scope1 : Scope  NumInputPorts=3
  Sum1 : Sum  Inputs=+-  SaturateOnIntegerOverflow=on  InputSameDT=on  OutDataTypeStr=Inherit: Same as first input
  Sum2 : Sum  Inputs=+-  SaturateOnIntegerOverflow=on  InputSameDT=on  OutDataTypeStr=Inherit: Same as first input
  Sum4 : Sum  SaturateOnIntegerOverflow=on  InputSameDT=on  OutDataTypeStr=Inherit: Same as first input
  Vf : Outport
  wires:
  Sum2/1 -> Dead Band1/1
  Dead Band1/1 -> Product3/1
  Droop_v/1 -> Product3/2
  Product3/1 -> Sum4/1
  Vref/1 -> Sum2/1
  Qpcc/1 -> Scope1/3, Sum1/2
  Sum1/1 -> PI1/1
  PI1/1 -> Scope1/1, Vf/1
  fixed_Q/1 -> Sum4/2
  Sum4/1 -> Scope1/2, Sum1/1
  VPCC/1 -> Sum2/2

== system Feeder_IREQ_2012/Controllable load/Discrete 3-phase PLL-Driven  Positive-Sequence Active & Reactive Power/Discrete 3-phase PLL-Driven Positive-Sequence Fundamental Value ==
  note: Pierre Giroux, Gilbert Sybille
      | Power System Simulation Laboratory
      | IREQ, Hydro-Quebc
  note: Discrete 3-phase PLL-Driven Positive-Sequence Fundamental Value
  Freq : Inport
  Sin_Cos : Inport  Port=2  PortDimensions=2
  abc : Inport  Port=3  PortDimensions=3
  Cartesian to Polar : simulink_extras/Transformations/Cartesian to Polar
  Demux : Demux  Outputs=3
  Discrete Variable Frequency Mean value1 : Subsystem  mask(Discrete Variable-Frequency Mean Value){Finit=Finit, Fmin=Fmin, Vinit=Imag_Init, Ts=Ts}
      mask prompts: Finit "Initial frequency (Hz):"; Fmin "Minimum frequency (Hz):"; Vinit "Initial input (DC component):"; Ts "Sample time:"
      mask help:
      | This discrete block computes the mean value of the input signal (port In) over a running window of one cycle of a specified frequency (port Freq).
      |
      | For the first cycle of simulation (specified by the parameter "Initial frequency"), the output is held to the value of the  "Initial input" parameter.
      |
      | The value of the parameter "Minimum frequency" is used to determine the buffer size of the "Variable Transport Delay" block found inside this subsystem.
      mask init:
      | MaxDelay=1/Fmin+Ts;
      | power_initmask();
      settings: OpenFcn=power_openblockproxy();
  Discrete Variable Frequency Mean value2 : Subsystem  mask(Discrete Variable-Frequency Mean Value){Finit=Finit, Fmin=Fmin, Vinit=Real_Init, Ts=Ts}
      mask prompts: Finit "Initial frequency (Hz):"; Fmin "Minimum frequency (Hz):"; Vinit "Initial input (DC component):"; Ts "Sample time:"
      mask help:
      | This discrete block computes the mean value of the input signal (port In) over a running window of one cycle of a specified frequency (port Freq).
      |
      | For the first cycle of simulation (specified by the parameter "Initial frequency"), the output is held to the value of the  "Initial input" parameter.
      |
      | The value of the parameter "Minimum frequency" is used to determine the buffer size of the "Variable Transport Delay" block found inside this subsystem.
      mask init:
      | MaxDelay=1/Fmin+Ts;
      | power_initmask();
      settings: OpenFcn=power_openblockproxy();
  Rad->Deg. : Gain  Gain=180/pi  SaturateOnIntegerOverflow=on  OutDataTypeStr=Inherit: Same as input  ParamDataTypeStr=Inherit: Same as input
  Terminator : Terminator
  abc_to_dq0 Transformation : powerlib_extras/Measurements/abc_to_dq0 Transformation
  Mag : Outport
  Phase : Outport  Port=2
  wires:
  Sin_Cos/1 -> abc_to_dq0 Transformation/2
  Freq/1 -> Discrete Variable Frequency Mean value2/1(Freq), Discrete Variable Frequency Mean value1/1(Freq)
  Discrete Variable Frequency Mean value2/1(Mean) -> Cartesian to Polar/1  "Real"
  Rad->Deg./1 -> Phase/1
  Discrete Variable Frequency Mean value1/1(Mean) -> Cartesian to Polar/2  "Real"
  Demux/2 -> Discrete Variable Frequency Mean value1/2(In)
  Demux/1 -> Discrete Variable Frequency Mean value2/2(In)
  abc/1 -> abc_to_dq0 Transformation/1
  abc_to_dq0 Transformation/1 -> Demux/1
  Demux/3 -> Terminator/1
  Cartesian to Polar/1 -> Mag/1
  Cartesian to Polar/2 -> Rad->Deg./1
